simulink library "mech_planetary_vrlib"  (Simulink 7.1)
libraries: vrlib x1
settings Model: Creator=arnav  LastModifiedBy=batserve

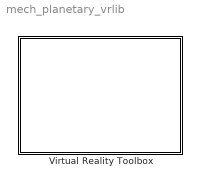
== system mech_planetary_vrlib ==
  Virtual Reality Toolbox : Subsystem  Orientation=left
      mask Display: disp(sprintf('Double-click to open\nVirtual Reality Toolbox viewer'))

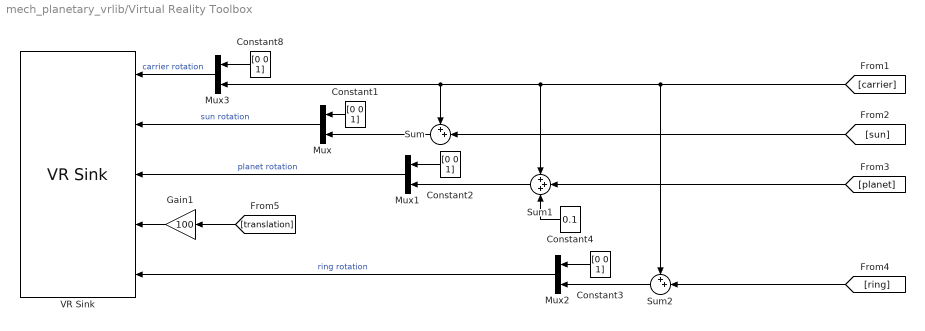
== system mech_planetary_vrlib/Virtual Reality Toolbox ==
  Constant{1..3,8} (4 alike) : Constant  Orientation=left  Value=[0 0 1]  OutDataType=sfix(16)  OutScaling=2^0
  Constant4 : Constant  Orientation=left  Value=0.1  OutDataType=sfix(16)  OutScaling=2^0
  Gain1 : Gain  Orientation=left  Gain=100  ParameterDataType=sfix(16)  ParameterScaling=2^0  OutDataType=sfix(16)  OutScaling=2^0  SaturateOnIntegerOverflow=on  OutDataTypeStr=Inherit: Same as input  ParamDataTypeStr=Inherit: Same as input
  Mux{,1..3} (4 alike) : Mux  Orientation=left  Inputs=2
  Sum : Sum  Orientation=left  Inputs=++|  OutDataType=sfix(16)  OutScaling=2^0  SaturateOnIntegerOverflow=on  InputSameDT=on  OutDataTypeStr=Inherit: Same as first input
  Sum1 : Sum  Orientation=left  Inputs=+++  OutDataType=sfix(16)  OutScaling=2^0  SaturateOnIntegerOverflow=on  InputSameDT=on  OutDataTypeStr=Inherit: Same as first input
  Sum2 : Sum  Orientation=left  Inputs=++|  OutDataType=sfix(16)  OutScaling=2^0  SaturateOnIntegerOverflow=on  InputSameDT=on  OutDataTypeStr=Inherit: Same as first input
  VR Sink : vrlib/VR Sink  Orientation=left  SampleTime=0.1  ViewEnable=on  RemoteChange=off  RemoteView=off  FieldsWritten=carrier.rotation#drum.rotation#planet.rotation#planet.translation#ring.rotation  WorldFileName=mech_planetary_world.wrl  WorldDescription=VR Planetary Gear Model  AutoView=off  FigureProperties={}
  wires:
  Constant4/1 -> Sum1/3
  [translation] -> Gain1/1
  Gain1/1 -> VR Sink/4
  [ring] -> Sum2/2
  Sum2/1 -> Mux2/2
  [planet] -> Sum1/2
  Sum1/1 -> Mux1/2
  [sun] -> Sum/2
  Sum/1 -> Mux/2
  Mux2/1 -> VR Sink/5  "ring rotation"
  Mux1/1 -> VR Sink/3  "planet rotation"
  Mux/1 -> VR Sink/2  "sun rotation"
  [carrier] -> Sum2/1, Sum1/1, Sum/1, Mux3/2
  Mux3/1 -> VR Sink/1  "carrier rotation"
  Constant3/1 -> Mux2/1
  Constant2/1 -> Mux1/1
  Constant1/1 -> Mux/1
  Constant8/1 -> Mux3/1
